simulink model "Lab7_E1"  (R2020b)
settings: Solver=VariableStepAuto  StartTime=0.0  StopTime=10  FixedStep=0  RelTol=1e-3
libraries: neural x28, simulink x2
(part 2 of 2)

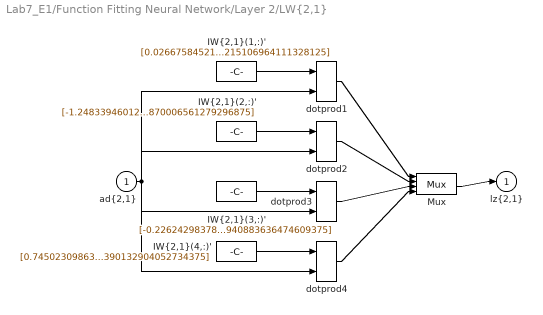
== system Lab7_E1/Function Fitting Neural Network/Layer 2/LW{2,1} ==
  "ad{2,1}" : Inport  PortDimensions=20
      mask Display: e = 0.06;c1 = [120 230 180]/255;c2 = ([120 230 180]+0)/(256+128);c3 = ([120 230 180]+128)/(256+128);patch([0 1 1 0],[0 0 1 1],c1);patch([0 1 1 1-e 1-e 0+e],[0 0 1 1-e 0+e 0+e],c2);patch([0 0 1 1-e 0+e 0+e],[0 1 1 1-e 1-e 0+e],c3);plot([0 1 1 0 0],[0 0 1 1 0]);
  "IW{2,1}(1,:)'" : Constant  Value=[0.026675845218452065576997256357572041451930999755859375;-0.10126845530414048390799308663190458901226520538330078125;-0.0250774330407973582157676872839147108606994152069091796875;-0.71488803256194077828666877394425682723522186279296875;0.319557664662871498961749239242635667324066162109375;-0.00102440618500659256888407622199110846850089728832244873046875;0.3700621055568635853205705643631517887115478515625;-0.06408429150791399020459238045077654533088207244873046875;0.00018732960077032882457818974142327306253719143569469451904296875;-0.055851218684562810301574842242189333774149417877197265625;-0.489743964242012719267904685693792998790740966796875;-1.5451652156928066261798448977060616016387939453125;0.1422457807015050368359965204945183359086513519287109375;-1.260541354612378928123916921322233974933624267578125;0.08665644082621011545786160468196612782776355743408203125;-0.020526927308309961262011711369268596172332763671875;0.58960770886592206441179087050841189920902252197265625;-0.51216331458412545085678857503808103501796722412109375;-0.281782284994048726201043564287829212844371795654296875;0.0649237297241876121223214113342692144215106964111328125]
      mask Display: e = 0.06;c1 = [120 150 230]/255;c2 = ([120 150 230]+0)/383;c3 = ([120 150 230]+128)/383;patch([0 1 1 0],[0 0 1 1],c1);patch([0 1 1 1-e 1-e 0+e],[0 0 1 1-e 0+e 0+e],c2);patch([0 0 1 1-e 0+e 0+e],[0 1 1 1-e 1-e 0+e],c3);plot([0 1 1 0 0],[0 0 1 1 0]);disp('weights');
  "IW{2,1}(2,:)'" : Constant  Value=[-1.2483394601278667845889458476449362933635711669921875;0.061577600872825259681331289129957440309226512908935546875;-0.037178833821612973509207478173266281373798847198486328125;-0.2347994466474962182989116854514577426016330718994140625;-0.261513705559294262759095772707951255142688751220703125;0.000712107873674910321799835788425525606726296246051788330078125;-0.468534969581737126276266280910931527614593505859375;2.084405122145275957024068702594377100467681884765625;5.48600874348734621438299086104706248079310171306133270263671875e-05;-0.12146406691951865119971643025564844720065593719482421875;0.08189763266721195034136826507165096700191497802734375;-0.607419180501031608088169377879239618778228759765625;0.2078743029588409896302181323335389606654644012451171875;1.0420520720940753545136203683796338737010955810546875;-0.278661361322785128269430288128205575048923492431640625;-0.11359101376757281542939637120070983655750751495361328125;-0.494454738448701747177693732737679965794086456298828125;0.50743632845860187075004432699643075466156005859375;-0.10306174665240853960401778977029607631266117095947265625;-0.09476794320342578348270734522884595207870006561279296875]
      mask Display: e = 0.06;c1 = [120 150 230]/255;c2 = ([120 150 230]+0)/383;c3 = ([120 150 230]+128)/383;patch([0 1 1 0],[0 0 1 1],c1);patch([0 1 1 1-e 1-e 0+e],[0 0 1 1-e 0+e 0+e],c2);patch([0 0 1 1-e 0+e 0+e],[0 1 1 1-e 1-e 0+e],c3);plot([0 1 1 0 0],[0 0 1 1 0]);disp('weights');
  "IW{2,1}(3,:)'" : Constant  Value=[-0.22624298378456375591127880397834815084934234619140625;0.036553569359838035401910616428722278214991092681884765625;0.09796419631980675390980906058757682330906391143798828125;0.3396400712636642449382406994118355214595794677734375;0.039187806194914076574065120439627207815647125244140625;-0.0017265489101011767709981103990912743029184639453887939453125;0.11679739520478461811681114568273187614977359771728515625;0.397035462196153876579529651280608959496021270751953125;-4.8657987957502476120759567213003293772999313659965991973876953125e-06;1.7026588341069828214102699348586611449718475341796875;0.40287125331111128812011656918912194669246673583984375;0.60248823230759729341343700070865452289581298828125;0.86645247636511657507440986591973342001438140869140625;-1.071057870902139885771475746878422796726226806640625;-0.83643065484039025303530934252194128930568695068359375;-0.1633256323942194609966094276387593708932399749755859375;1.81217007455159784257148203323595225811004638671875;1.6618230415820069989507601349032483994960784912109375;-0.242285819167607219259963358126697130501270294189453125;-0.49920417827785035225218734922236762940883636474609375]
      mask Display: e = 0.06;c1 = [120 150 230]/255;c2 = ([120 150 230]+0)/383;c3 = ([120 150 230]+128)/383;patch([0 1 1 0],[0 0 1 1],c1);patch([0 1 1 1-e 1-e 0+e],[0 0 1 1-e 0+e 0+e],c2);patch([0 0 1 1-e 0+e 0+e],[0 1 1 1-e 1-e 0+e],c3);plot([0 1 1 0 0],[0 0 1 1 0]);disp('weights');
  "IW{2,1}(4,:)'" : Constant  Value=[0.74502309863869131678626445136615075170993804931640625;0.258051567249830193784276843871339224278926849365234375;-0.2392513132406336173740868389359093271195888519287109375;-1.4030763609083101162156026475713588297367095947265625;-0.9475939854598995903955938047147355973720550537109375;0.00177846965778486539207225991532368425396271049976348876953125;1.1727827559856027761497898609377443790435791015625;-1.2819349917556761564441103473654948174953460693359375;-2.700644901423081438766003736784426791928126476705074310302734375e-05;-1.907060044810022336747579174698330461978912353515625;-1.296515758775823368154078707448206841945648193359375;0.52730324125856398165268501543323509395122528076171875;1.236642226040246317353421545703895390033721923828125;2.60859633971998494672561719198711216449737548828125;-2.018727558659665799467575197922997176647186279296875;-1.121826676964665647773244927520863711833953857421875;0.317947021115084493825264644328854046761989593505859375;2.535993033183476796921240747906267642974853515625;-1.4741514714151191522972794700763188302516937255859375;-0.49515108988049882920989830381586216390132904052734375]
      mask Display: e = 0.06;c1 = [120 150 230]/255;c2 = ([120 150 230]+0)/383;c3 = ([120 150 230]+128)/383;patch([0 1 1 0],[0 0 1 1],c1);patch([0 1 1 1-e 1-e 0+e],[0 0 1 1-e 0+e 0+e],c2);patch([0 0 1 1-e 0+e 0+e],[0 1 1 1-e 1-e 0+e],c3);plot([0 1 1 0 0],[0 0 1 1 0]);disp('weights');
  Mux : Mux
      mask Display: e = 0.06;c1 = [120 150 230]/255;c2 = ([120 150 230]+0)/383;c3 = ([120 150 230]+128)/383;patch([0 1 1 0],[0 0 1 1],c1);patch([0 1 1 1-e 1-e 0+e],[0 0 1 1-e 0+e 0+e],c2);patch([0 0 1 1-e 0+e 0+e],[0 1 1 1-e 1-e 0+e],c3);plot([0 1 1 0 0],[0 0 1 1 0]);disp('Mux');
  dotprod{1..4} (4 alike) : neural/Weight Functions/dotprod
  "lz{2,1}" : Outport
      mask Display: e = 0.06;c1 = [120 230 180]/255;c2 = ([120 230 180]+0)/(256+128);c3 = ([120 230 180]+128)/(256+128);patch([0 1 1 0],[0 0 1 1],c1);patch([0 1 1 1-e 1-e 0+e],[0 0 1 1-e 0+e 0+e],c2);patch([0 0 1 1-e 0+e 0+e],[0 1 1 1-e 1-e 0+e],c3);plot([0 1 1 0 0],[0 0 1 1 0]);
  wires:
  "IW{2,1}(1,:)'"/1 -> dotprod1/1
  "ad{2,1}"/1 -> dotprod1/2, dotprod2/2, dotprod3/2, dotprod4/2
  dotprod1/1 -> Mux/1
  "IW{2,1}(2,:)'"/1 -> dotprod2/1
  dotprod2/1 -> Mux/2
  "IW{2,1}(3,:)'"/1 -> dotprod3/1
  dotprod3/1 -> Mux/3
  "IW{2,1}(4,:)'"/1 -> dotprod4/1
  dotprod4/1 -> Mux/4
  Mux/1 -> "lz{2,1}"/1

== matlab function Lab7_E1/Subsystem/MATLAB Function ==
  data: u input; q1 input; x1_dot output; q2 input; x2_dot output; q1_dot input; q2_dot input
function [x1_dot, x2_dot] = fcn(u, q1, q2, q1_dot, q2_dot)
    x1 = [q1 ; q2];
    x2 = [q1_dot ; q2_dot];

    a1 = 200.01;
    a2 = 23.5;
    a3 = 122.5;
    a4 = 25;
    b1 = 784.8;
    b2 = 245.25;
    C = a4 * sin(q2) * [-q2_dot -(q1_dot + q2_dot) ; q1_dot  0];
    g = [b1 * cos(q1) + b2 * cos(q1 + q2) ; b2 * cos(q1 + q2)];
    M = [a1 + 2 * a4 * cos(q2) a2 + a4 * cos(q2) ; a2 + a4 * cos(q2) a3];
    D = 0;
    
    x1_dot = x2;
    x2_dot = M^-1 * (u - C * x2 - D * x2 - g);

== matlab function Lab7_E1/Subsystem2/MATLAB Function ==
  data: u input; q1 input; x1_dot output; q2 input; x2_dot output; q1_dot input; q2_dot input
function [x1_dot, x2_dot] = fcn(u, q1, q2, q1_dot, q2_dot)
    x1 = [q1 ; q2];
    x2 = [q1_dot ; q2_dot];

    a1 = 200.01;
    a2 = 23.5;
    a3 = 122.5;
    a4 = 25;
    b1 = 784.8;
    b2 = 245.25;
    C = a4 * sin(q2) * [-q2_dot -(q1_dot + q2_dot) ; q1_dot  0];
    g = [b1 * cos(q1) + b2 * cos(q1 + q2) ; b2 * cos(q1 + q2)];
    M = [a1 + 2 * a4 * cos(q2) a2 + a4 * cos(q2) ; a2 + a4 * cos(q2) a3];
    D = 0;
    
    x1_dot = x2;
    x2_dot = M^-1 * (u - C * x2 - D * x2 - g);
